simulink model "Pendulo_LQR"  (R2023b)
settings: Solver=ode15s  StartTime=0.0  StopTime=50  MaxStep=0.06  RelTol=1e-3
undefined symbols (not defined in the file): b, g, K, L, M, m
libraries: simulink x4
settings Model: Creator=Usuario  LastModifiedBy=Usuario

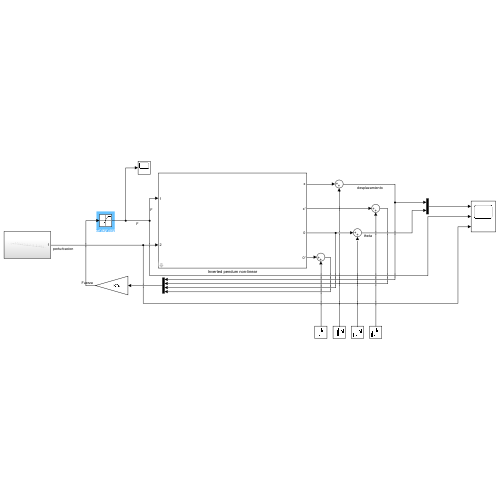
[thumbnail: Simulink's stored preview of the top-level diagram]
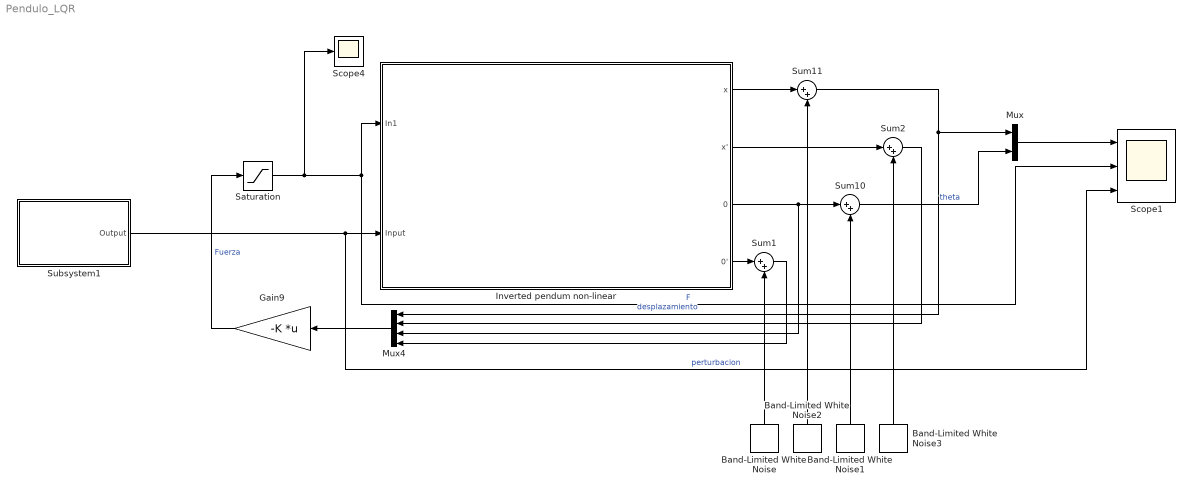
== system Pendulo_LQR ==
  Band-Limited White Noise : simulink/Sources/Band-Limited White Noise  Cov=[0.00001]  Ts=0.05  seed=[23341]
  Band-Limited White Noise1 : simulink/Sources/Band-Limited White Noise  Cov=[0.00001]  Ts=0.02  seed=[233]
  Band-Limited White Noise2 : simulink/Sources/Band-Limited White Noise  Cov=[0.00001]  Ts=0.03  seed=[341]
  Band-Limited White Noise3 : simulink/Sources/Band-Limited White Noise  Cov=[0.00001]  Ts=0.01  seed=[2341]
  Gain9 : Gain  Gain=-K  Multiplication=Matrix(K*u)
  Inverted pendum non-linear : Subsystem  mask{M_=M, L=L, g=g, angulo=0.2, m=m, b=b}
      mask prompts: M_ "M"; angulo "angulo inicial"
  Mux : Mux  Inputs=2
  Mux4 : Mux
  Saturation : Saturate  UpperLimit=10  LowerLimit=-10
  Scope1 : Scope  NumInputPorts=3
  Scope4 : Scope
  Subsystem1 : Subsystem
  Sum{1..2,10..11} (4 alike) : Sum  Inputs=|++
  wires:
  Mux4/1 -> Gain9/1
  Inverted pendum non-linear/2(x') -> Sum2/1
  Inverted pendum non-linear/4(0') -> Sum1/1
  Inverted pendum non-linear/3(0) -> Sum10/1, Mux4/3
  Gain9/1 -> Saturation/1  "Fuerza"
  Inverted pendum non-linear/1(x) -> Sum11/1
  Sum11/1 -> Mux/1, Mux4/1  "desplazamiento"
  Mux/1 -> Scope1/1
  Sum10/1 -> Mux/2  "theta"
  Band-Limited White Noise2/1 -> Sum11/2
  Band-Limited White Noise1/1 -> Sum10/2
  Sum1/1 -> Mux4/4
  Band-Limited White Noise/1 -> Sum1/2
  Sum2/1 -> Mux4/2
  Band-Limited White Noise3/1 -> Sum2/2
  Subsystem1/1(Output) -> Inverted pendum non-linear/2(Input), Scope1/3  "perturbacion"
  Saturation/1 -> Scope4/1, Scope1/2, Inverted pendum non-linear/1(In1)  "F"

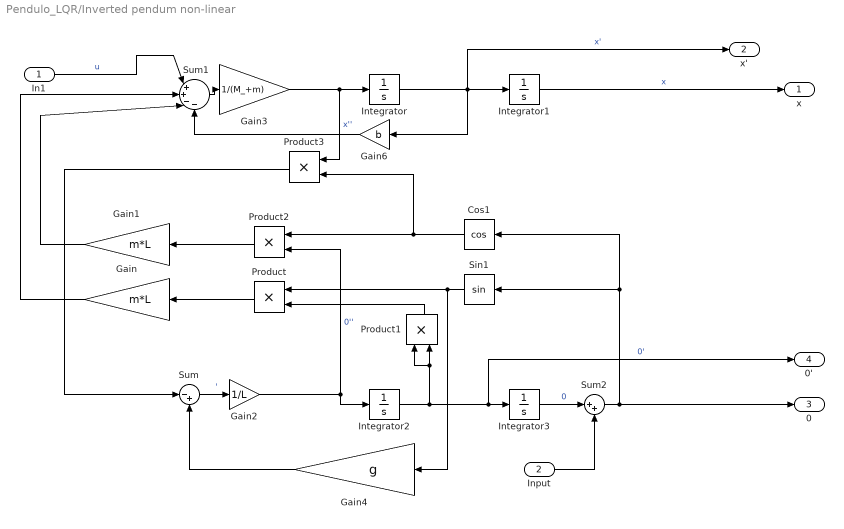
== system Pendulo_LQR/Inverted pendum non-linear ==
  In1 : Inport
  Input : Inport  Port=2
  Cos1 : Trigonometry  Operator=cos
  Gain : Gain  Gain=m*L
  Gain1 : Gain  Gain=m*L
  Gain2 : Gain  Gain=1/L
  Gain3 : Gain  Gain=1/(M_+m)
  Gain4 : Gain  Gain=g
  Gain6 : Gain  Gain=b
  Integrator : Integrator
  Integrator1 : Integrator
  Integrator2 : Integrator
  Integrator3 : Integrator  InitialCondition=angulo
  Product{,1..3} (4 alike) : Product
  Sin1 : Trigonometry
  Sum : Sum  Inputs=|-+
  Sum1 : Sum  Inputs=|++--
  Sum2 : Sum  Inputs=|++
  x : Outport
  x' : Outport  Port=2
  0 : Outport  Port=3
  0' : Outport  Port=4
  wires:
  Integrator/1 -> Gain6/1, Integrator1/1, x'/1  "x'"
  Integrator2/1 -> Product1/1, Product1/2, 0'/1, Integrator3/1  "0'"
  Integrator1/1 -> x/1  "x"
  Integrator3/1 -> Sum2/1  "0"
  Cos1/1 -> Product3/2, Product2/1
  Sin1/1 -> Gain4/1, Product/1
  Product1/1 -> Product/2
  Product/1 -> Gain/1
  Product2/1 -> Gain1/1
  Gain/1 -> Sum1/2
  Gain1/1 -> Sum1/3
  Product3/1 -> Sum/1
  Gain4/1 -> Sum/2
  Sum1/1 -> Gain3/1
  Gain3/1 -> Product3/1, Integrator/1  "x''"
  In1/1 -> Sum1/1  "u"
  Sum/1 -> Gain2/1  "'"
  Gain2/1 -> Integrator2/1, Product2/2  "0''"
  Sum2/1 -> Sin1/1, Cos1/1, 0/1
  Input/1 -> Sum2/2
  Gain6/1 -> Sum1/4

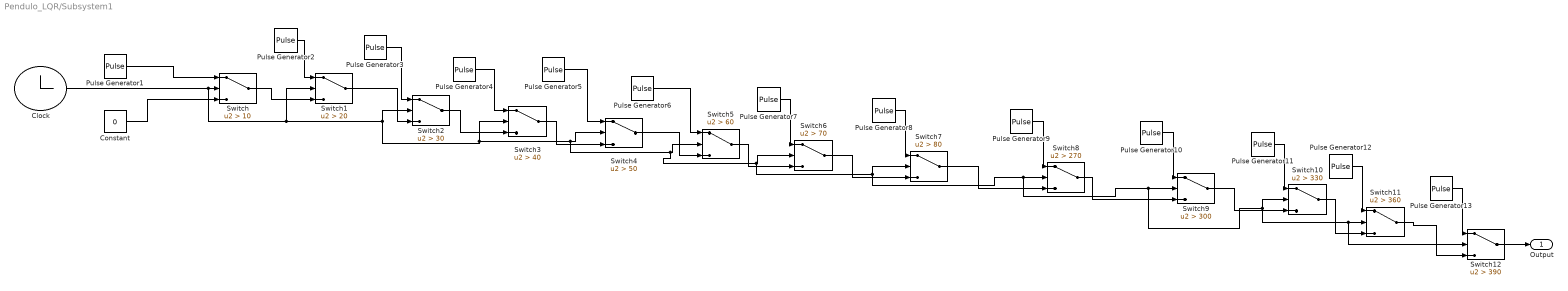
== system Pendulo_LQR/Subsystem1 ==
  Clock : Clock
  Constant : Constant  Value=0
  Pulse Generator1 : DiscretePulseGenerator  PulseType=Time based  Amplitude=0.1  Period=30  PulseWidth=2  PhaseDelay=11
  Pulse Generator10 : DiscretePulseGenerator  PulseType=Time based  Amplitude=2.1  Period=30  PulseWidth=50  PhaseDelay=300
  Pulse Generator11 : DiscretePulseGenerator  PulseType=Time based  Amplitude=2.3  Period=30  PulseWidth=50  PhaseDelay=330
  Pulse Generator12 : DiscretePulseGenerator  PulseType=Time based  Amplitude=2.5  Period=30  PulseWidth=50  PhaseDelay=360
  Pulse Generator13 : DiscretePulseGenerator  PulseType=Time based  Amplitude=2.7  Period=30  PulseWidth=50  PhaseDelay=390
  Pulse Generator2 : DiscretePulseGenerator  PulseType=Time based  Amplitude=0.2  Period=30  PhaseDelay=21
  Pulse Generator3 : DiscretePulseGenerator  PulseType=Time based  Amplitude=0.3  Period=30  PhaseDelay=31
  Pulse Generator4 : DiscretePulseGenerator  PulseType=Time based  Amplitude=0.4  Period=30  PhaseDelay=41
  Pulse Generator5 : DiscretePulseGenerator  PulseType=Time based  Amplitude=0.5  Period=30  PhaseDelay=51
  Pulse Generator6 : DiscretePulseGenerator  PulseType=Time based  Amplitude=0.6  Period=30  PhaseDelay=61
  Pulse Generator7 : DiscretePulseGenerator  PulseType=Time based  Amplitude=0.7  Period=30  PhaseDelay=71
  Pulse Generator8 : DiscretePulseGenerator  PulseType=Time based  Amplitude=0.8  Period=30  PhaseDelay=81
  Pulse Generator9 : DiscretePulseGenerator  PulseType=Time based  Amplitude=1.9  Period=30  PulseWidth=50  PhaseDelay=270
  Switch : Switch  Criteria=u2 > Threshold  Threshold=10  SaturateOnIntegerOverflow=off  InputSameDT=off
  Switch1 : Switch  Criteria=u2 > Threshold  Threshold=20  SaturateOnIntegerOverflow=off  InputSameDT=off
  Switch10 : Switch  Criteria=u2 > Threshold  Threshold=330  SaturateOnIntegerOverflow=off  InputSameDT=off
  Switch11 : Switch  Criteria=u2 > Threshold  Threshold=360  SaturateOnIntegerOverflow=off  InputSameDT=off
  Switch12 : Switch  Criteria=u2 > Threshold  Threshold=390  SaturateOnIntegerOverflow=off  InputSameDT=off
  Switch2 : Switch  Criteria=u2 > Threshold  Threshold=30  SaturateOnIntegerOverflow=off  InputSameDT=off
  Switch3 : Switch  Criteria=u2 > Threshold  Threshold=40  SaturateOnIntegerOverflow=off  InputSameDT=off
  Switch4 : Switch  Criteria=u2 > Threshold  Threshold=50  SaturateOnIntegerOverflow=off  InputSameDT=off
  Switch5 : Switch  Criteria=u2 > Threshold  Threshold=60  SaturateOnIntegerOverflow=off  InputSameDT=off
  Switch6 : Switch  Criteria=u2 > Threshold  Threshold=70  SaturateOnIntegerOverflow=off  InputSameDT=off
  Switch7 : Switch  Criteria=u2 > Threshold  Threshold=80  SaturateOnIntegerOverflow=off  InputSameDT=off
  Switch8 : Switch  Criteria=u2 > Threshold  Threshold=270  SaturateOnIntegerOverflow=off  InputSameDT=off
  Switch9 : Switch  Criteria=u2 > Threshold  Threshold=300  SaturateOnIntegerOverflow=off  InputSameDT=off
  Output : Outport
  wires:
  Pulse Generator1/1 -> Switch/1
  Constant/1 -> Switch/3
  Switch/1 -> Switch1/3
  Switch1/1 -> Switch2/3
  Pulse Generator3/1 -> Switch2/1
  Pulse Generator2/1 -> Switch1/1
  Pulse Generator4/1 -> Switch3/1
  Switch2/1 -> Switch3/3
  Pulse Generator5/1 -> Switch4/1
  Switch3/1 -> Switch4/3
  Pulse Generator6/1 -> Switch5/1
  Switch4/1 -> Switch5/3
  Pulse Generator7/1 -> Switch6/1
  Switch5/1 -> Switch6/3
  Pulse Generator8/1 -> Switch7/1
  Pulse Generator9/1 -> Switch8/1
  Switch7/1 -> Switch8/3
  Switch8/1 -> Switch9/3
  Pulse Generator10/1 -> Switch9/1
  Switch6/1 -> Switch7/3
  Pulse Generator11/1 -> Switch10/1
  Switch9/1 -> Switch10/3
  Switch10/1 -> Switch11/3
  Pulse Generator12/1 -> Switch11/1
  Pulse Generator13/1 -> Switch12/1
  Switch12/1 -> Output/1
  Clock/1 -> Switch3/2, Switch7/2, Switch8/2, Switch10/2, Switch12/2, Switch11/2, Switch9/2, Switch6/2, Switch5/2, Switch4/2, Switch2/2, Switch1/2, Switch/2
  Switch11/1 -> Switch12/3
